simulink model "bh_6dof_quat_integrate"  (R2019b)
settings: Solver=ode45  StartTime=0.0  StopTime=200  FixedStep=0.001  EnableMultiTasking=on
undefined symbols (not defined in the file or in its folder): P_elec, P_mot, P_one_prop, P_rot, P_veh, sigbuilder_block
libraries: bh_6dof_LIBRARY x23, simulink_extras x20, simulink x16
(part 1 of 3)
settings Model: Creator=bhorton  LastModifiedBy=bhorton
settings SolverCC: ZeroCrossAlgorithm=Adaptive  SolverOrder=4
settings DataIOCC: SaveOutput=off  SignalLogging=off  DSMLogging=off  VisualizeSimOutput=off  SaveTime=off  ReturnWorkspaceOutputs=off
settings OptimizationCC: LifeSpan=inf
settings DebuggingCC: AllowSymbolicDim=off  SFUnexpectedBacktrackingDiag=warning  SFNoUnconditionalDefaultTransitionDiag=warning  ArithmeticOperatorsInVariantConditions=warning
settings ModelReferenceCC: PropagateSignalLabelsOutOfModel=off
settings SFSimCC: SimUseLocalCustomCode=off  CustomCodeUndefinedFunction=UseInterfaceOnly
settings RTWCC: RTWUseLocalCustomCode=off
settings CodeAppCC: StateflowObjectComments=on
settings GRTTargetCC: TargetLangStandard=C89/C90 (ANSI)
settings ConfigComp: CovMetricSettings=dw  CovHtmlReporting=on  CovSaveCumulativeToWorkspaceVar=on  CovSaveSingleToWorkspaceVar=on  CovExternalEMLEnable=off

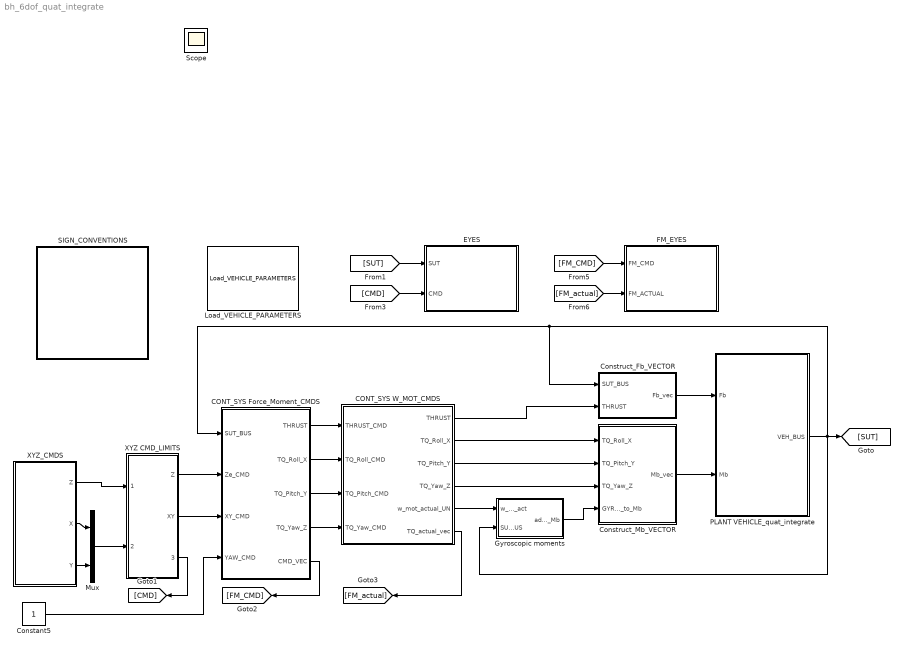
== system bh_6dof_quat_integrate ==
  CONT_SYS Force_Moment_CMDS : Subsystem
  CONT_SYS W_MOT_CMDS : Subsystem
  Constant5 : Constant
  Construct_Fb_VECTOR : Subsystem
  Construct_Mb_VECTOR : Subsystem
  EYES : Subsystem
      mask Display: image('bh_PIC_SCOPE.jpg');
  FM_EYES : Subsystem
      mask Display: image('bh_PIC_SCOPE.jpg');
  Gyroscopic moments : Subsystem
  Load_VEHICLE_PARAMETERS : bh_6dof_LIBRARY/MODELS/Load_VEHICLE_PARAMETERS  SystemSampleTime=-1  Latency=0  AutoFrameSizeCalculation=off
  Mux : Mux  Inputs=2
  PLANT VEHICLE_quat_integrate : Subsystem
  SIGN_CONVENTIONS : Subsystem
  XYZ CMD_LIMITS : Subsystem
  XYZ_CMDS : Subsystem  Tag=STV Subsys  LoadFcn=sigbuilder_block('load');  StartFcn=sigbuilder_block('start');  StopFcn=sigbuilder_block('stop');  ClipboardFcn=sigbuilder_block('clipboard');  mask(Sigbuilder block){tuvar=[0:10]}
      mask help: Simulink:masks:SigbuilderBlock_MD
      mask init:
      | if ~strcmp(get_param(bdroot(gcbh),'SimulationStatus'),'stopped') tuvar = sigbuilder_block('maskInit'); end
      settings: CopyFcn=sigbuilder_block('copy');  DeleteFcn=sigbuilder_block('delete');  ModelCloseFcn=sigbuilder_block('modelClose');  PreSaveFcn=sigbuilder_block('preSave');  PauseFcn=sigbuilder_block('pause');  ContinueFcn=sigbuilder_block('continue');  NameChangeFcn=sigbuilder_block('namechange');  OpenFcn=sigbuilder_block('open',[189 32.25 551.25 400.5 ]);  CloseFcn=sigbuilder_block('close');
      mask Display: plot(0, 0, 100, 100,[2, 2, 32, 32, 2], [68, 8, 8, 68, 68],[32, 2], [38, 38], [32, 19, 2],[53, 60, 44], [32, 17, 17, 2],[16, 16, 31, 31]);txt = getActiveGroup(gcbh);text(2, 100, txt,'verticalAlignment', 'top');
  Scope : Scope
  wires:
  Construct_Fb_VECTOR/1(Fb_vec) -> PLANT VEHICLE_quat_integrate/1(Fb)
  Construct_Mb_VECTOR/1(Mb_vec) -> PLANT VEHICLE_quat_integrate/2(Mb)
  CONT_SYS Force_Moment_CMDS/1(THRUST) -> CONT_SYS W_MOT_CMDS/1(THRUST_CMD)
  Constant5/1 -> CONT_SYS Force_Moment_CMDS/4(YAW_CMD)
  XYZ_CMDS/1(Z) -> XYZ CMD_LIMITS/1(Z_CMD)
  [SUT] -> EYES/1(SUT)
  [CMD] -> EYES/2(CMD)
  XYZ CMD_LIMITS/3(CMD_BUS) -> [CMD]
  XYZ CMD_LIMITS/2(XY) -> CONT_SYS Force_Moment_CMDS/3(XY_CMD)
  XYZ CMD_LIMITS/1(Z) -> CONT_SYS Force_Moment_CMDS/2(Ze_CMD)
  Mux/1 -> XYZ CMD_LIMITS/2(XY_CMD)
  XYZ_CMDS/3(Y) -> Mux/2
  XYZ_CMDS/2(X) -> Mux/1
  CONT_SYS W_MOT_CMDS/1(THRUST) -> Construct_Fb_VECTOR/2(THRUST)
  CONT_SYS W_MOT_CMDS/2(TQ_Roll_X) -> Construct_Mb_VECTOR/1(TQ_Roll_X)
  CONT_SYS W_MOT_CMDS/3(TQ_Pitch_Y) -> Construct_Mb_VECTOR/2(TQ_Pitch_Y)
  CONT_SYS W_MOT_CMDS/4(TQ_Yaw_Z) -> Construct_Mb_VECTOR/3(TQ_Yaw_Z)
  CONT_SYS W_MOT_CMDS/6(TQ_actual_vec) -> [FM_actual]
  [FM_CMD] -> FM_EYES/1(FM_CMD)
  [FM_actual] -> FM_EYES/2(FM_ACTUAL)
  PLANT VEHICLE_quat_integrate/1(VEH_BUS) -> Gyroscopic moments/2(SUT_BUS), Construct_Fb_VECTOR/1(SUT_BUS), CONT_SYS Force_Moment_CMDS/1(SUT_BUS), [SUT]
  Gyroscopic moments/1(add_to_Mb) -> Construct_Mb_VECTOR/4(GYRO_add_to_Mb)
  CONT_SYS W_MOT_CMDS/5(w_mot_actual_UN) -> Gyroscopic moments/1(w_mot_act)
  CONT_SYS Force_Moment_CMDS/2(TQ_Roll_X) -> CONT_SYS W_MOT_CMDS/2(TQ_Roll_CMD)
  CONT_SYS Force_Moment_CMDS/3(TQ_Pitch_Y) -> CONT_SYS W_MOT_CMDS/3(TQ_Pitch_CMD)
  CONT_SYS Force_Moment_CMDS/4(TQ_Yaw_Z) -> CONT_SYS W_MOT_CMDS/4(TQ_Yaw_CMD)
  CONT_SYS Force_Moment_CMDS/5(CMD_VEC) -> [FM_CMD]

== system bh_6dof_quat_integrate/CONT_SYS Force_Moment_CMDS ==
  SUT_BUS : Inport
  Ze_CMD : Inport  Port=2
  XY_CMD : Inport  Port=3
  YAW_CMD : Inport  Port=4
  Constant3 : Constant  Value=P_veh.mass
  FM_CMD_LIMITS : Subsystem
  Gain : Gain  Gain=9.81
  PITCH_and_ROLL_CONT : Subsystem
  Sum2 : Sum  Inputs=++|
  YAW_CONT : Subsystem
  Z_CONT : Subsystem
  THRUST : Outport
  TQ_Roll_X : Outport  Port=2
  TQ_Pitch_Y : Outport  Port=3
  TQ_Yaw_Z : Outport  Port=4
  CMD_VEC : Outport  Port=5
  wires:
  SUT_BUS/1 -> YAW_CONT/2(SUT_BUS), PITCH_and_ROLL_CONT/2(SUT_BUS), Z_CONT/2(SUT_BUS)
  Ze_CMD/1 -> Z_CONT/1(Ze_CMD)
  XY_CMD/1 -> PITCH_and_ROLL_CONT/1(XY_CMD)
  YAW_CMD/1 -> YAW_CONT/1(Yaw_CMD)
  Z_CONT/1(THRUST) -> Sum2/2
  PITCH_and_ROLL_CONT/1(TQ_Roll) -> FM_CMD_LIMITS/2(TQ_Roll)
  PITCH_and_ROLL_CONT/2(TQ_Pitch) -> FM_CMD_LIMITS/3(TQ_Pitch)
  Sum2/1 -> FM_CMD_LIMITS/1(T_CMD)
  YAW_CONT/1(TQ_Yaw) -> FM_CMD_LIMITS/4(TQ_Yaw)
  FM_CMD_LIMITS/1(THRUST) -> THRUST/1
  FM_CMD_LIMITS/2(TQ_Roll_X) -> TQ_Roll_X/1
  FM_CMD_LIMITS/3(TQ_Pitch_Y) -> TQ_Pitch_Y/1
  FM_CMD_LIMITS/4(TQ_Yaw_Z) -> TQ_Yaw_Z/1
  FM_CMD_LIMITS/5(CMD_VEC) -> CMD_VEC/1
  Gain/1 -> Sum2/1
  Constant3/1 -> Gain/1

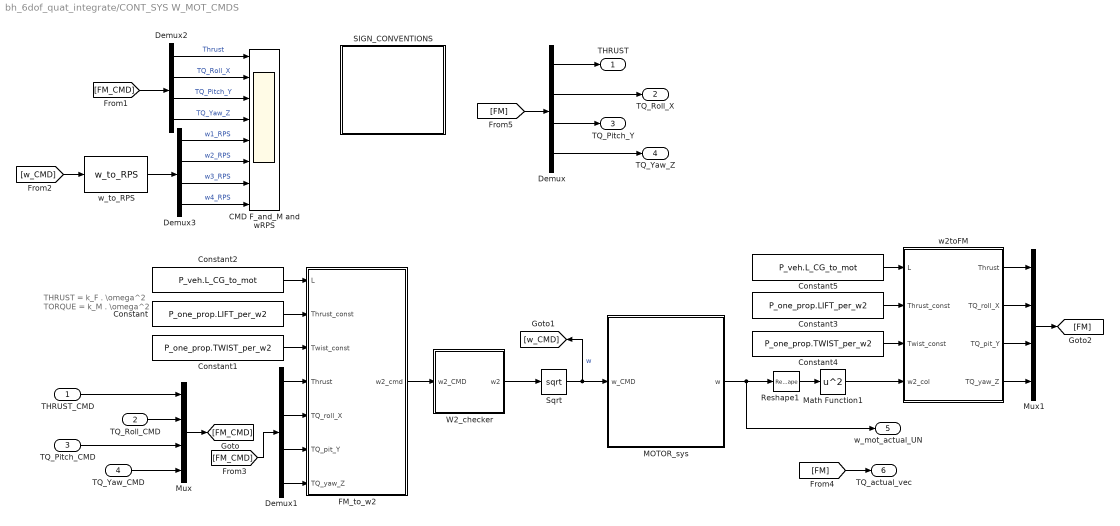
== system bh_6dof_quat_integrate/CONT_SYS W_MOT_CMDS ==
  note: THRUST = k_F . \omega^2
      |
      | TORQUE = k_M . \omega^2
  THRUST_CMD : Inport
  TQ_Roll_CMD : Inport  Port=2
  TQ_Pitch_CMD : Inport  Port=3
  TQ_Yaw_CMD : Inport  Port=4
  CMD F_and_M and wRPS : Scope  NumInputPorts=8
  Constant : Constant  Value=P_one_prop.LIFT_per_w2
  Constant1 : Constant  Value=P_one_prop.TWIST_per_w2
  Constant2 : Constant  Value=P_veh.L_CG_to_mot
  Constant3 : Constant  Value=P_one_prop.LIFT_per_w2
  Constant4 : Constant  Value=P_one_prop.TWIST_per_w2
  Constant5 : Constant  Value=P_veh.L_CG_to_mot
  Demux{,1..3} (4 alike) : Demux
  FM_to_w2 : MATLAB Function  TreatAsAtomicUnit=on
  MOTOR_sys : Subsystem
      mask Display: image('bh_PIC_MOTOR.jpg');
  Math Function1 : Math  Operator=square  SaturateOnIntegerOverflow=on
  Mux : Mux
  Mux1 : Mux
  Reshape1 : Reshape  OutputDimensionality=Column vector (2-D)
  SIGN_CONVENTIONS : Subsystem
  Sqrt : Sqrt  SaturateOnIntegerOverflow=on
  W2_checker : Subsystem
  w2toFM : MATLAB Function  TreatAsAtomicUnit=on
  w_to_RPS : bh_6dof_LIBRARY/MODELS/w_to_RPS  SystemSampleTime=-1  Latency=0  AutoFrameSizeCalculation=off
  THRUST : Outport
  TQ_Roll_X : Outport  Port=2
  TQ_Pitch_Y : Outport  Port=3
  TQ_Yaw_Z : Outport  Port=4
  w_mot_actual_UN : Outport  Port=5
  TQ_actual_vec : Outport  Port=6
  wires:
  Constant1/1 -> FM_to_w2/3(Twist_const)
  Constant/1 -> FM_to_w2/2(Thrust_const)
  Constant2/1 -> FM_to_w2/1(L)
  FM_to_w2/1(w2_cmd) -> W2_checker/1(w2_CMD)
  Sqrt/1 -> MOTOR_sys/1(w_CMD), [w_CMD]  "w"
  W2_checker/1(w2) -> Sqrt/1
  Demux1/1 -> FM_to_w2/4(Thrust)
  Demux1/2 -> FM_to_w2/5(TQ_roll_X)
  Demux1/3 -> FM_to_w2/6(TQ_pit_Y)
  Demux1/4 -> FM_to_w2/7(TQ_yaw_Z)
  THRUST_CMD/1 -> Mux/1
  TQ_Roll_CMD/1 -> Mux/2
  TQ_Pitch_CMD/1 -> Mux/3
  TQ_Yaw_CMD/1 -> Mux/4
  Mux/1 -> [FM_CMD]
  [FM_CMD] -> Demux1/1
  Demux2/1 -> CMD F_and_M and wRPS/1  "Thrust"
  Demux2/2 -> CMD F_and_M and wRPS/2  "TQ_Roll_X"
  Demux2/3 -> CMD F_and_M and wRPS/3  "TQ_Pitch_Y"
  Demux2/4 -> CMD F_and_M and wRPS/4  "TQ_Yaw_Z"
  Demux3/2 -> CMD F_and_M and wRPS/6  "w2_RPS"
  Demux3/1 -> CMD F_and_M and wRPS/5  "w1_RPS"
  Demux3/4 -> CMD F_and_M and wRPS/8  "w4_RPS"
  Demux3/3 -> CMD F_and_M and wRPS/7  "w3_RPS"
  [FM_CMD] -> Demux2/1
  w_to_RPS/1 -> Demux3/1
  [w_CMD] -> w_to_RPS/1
  Constant3/1 -> w2toFM/2(Thrust_const)
  Constant4/1 -> w2toFM/3(Twist_const)
  Constant5/1 -> w2toFM/1(L)
  w2toFM/1(Thrust) -> Mux1/1
  w2toFM/2(TQ_roll_X) -> Mux1/2
  w2toFM/3(TQ_pit_Y) -> Mux1/3
  w2toFM/4(TQ_yaw_Z) -> Mux1/4
  Mux1/1 -> [FM]
  Demux/1 -> THRUST/1
  Demux/2 -> TQ_Roll_X/1
  Demux/4 -> TQ_Yaw_Z/1
  Demux/3 -> TQ_Pitch_Y/1
  [FM] -> Demux/1
  Reshape1/1 -> Math Function1/1
  Math Function1/1 -> w2toFM/4(w2_col)
  [FM] -> TQ_actual_vec/1
  MOTOR_sys/1(w) -> Reshape1/1, w_mot_actual_UN/1

== system bh_6dof_quat_integrate/Construct_Fb_VECTOR ==
  SUT_BUS : Inport
  THRUST : Inport  Port=2
  Bus Selector1 : BusSelector  OutputSignals=DCM_bRg
  Constant1 : Constant  Value=0
  Gravity_G_to_B : Subsystem
  Mux : Mux  Inputs=3
  Reshape : Reshape  OutputDimensionality=Column vector (2-D)
  Sum : Sum  Inputs=++|
  Fb_vec : Outport
  wires:
  Mux/1 -> Reshape/1
  Sum/1 -> Fb_vec/1
  SUT_BUS/1 -> Bus Selector1/1
  THRUST/1 -> Mux/3  "THRUST"
  Constant1/1 -> Mux/2, Mux/1
  Bus Selector1/1 -> Gravity_G_to_B/1(bRg)  "<DCM_bRg>"
  Gravity_G_to_B/1(Fb_gravity) -> Sum/1
  Reshape/1 -> Sum/2

== system bh_6dof_quat_integrate/Construct_Mb_VECTOR ==
  TQ_Roll_X : Inport
  TQ_Pitch_Y : Inport  Port=2
  TQ_Yaw_Z : Inport  Port=3
  GYRO_add_to_Mb : Inport  Port=4
  Mux1 : Mux  Inputs=3
  Reshape : Reshape  OutputDimensionality=Column vector (2-D)
  Reshape1 : Reshape  OutputDimensionality=Column vector (2-D)
  Sum : Sum  Inputs=+|+
  Mb_vec : Outport
  wires:
  TQ_Yaw_Z/1 -> Mux1/3
  TQ_Pitch_Y/1 -> Mux1/2
  TQ_Roll_X/1 -> Mux1/1
  Mux1/1 -> Reshape/1
  Sum/1 -> Reshape1/1
  Reshape/1 -> Sum/1
  GYRO_add_to_Mb/1 -> Sum/2
  Reshape1/1 -> Mb_vec/1

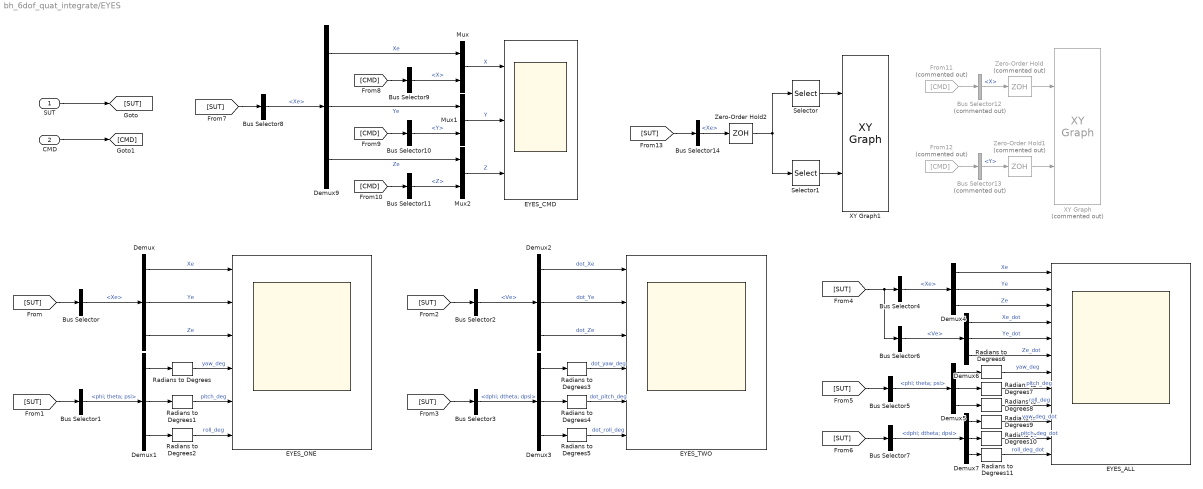
== system bh_6dof_quat_integrate/EYES ==
  SUT : Inport
  CMD : Inport  Port=2
  Bus Selector{,4,8,14} (4 alike) : BusSelector  OutputSignals=Xe
  Bus Selector1 : BusSelector  OutputSignals=phi; theta; psi
  Bus Selector10 : BusSelector  OutputSignals=Y
  Bus Selector11 : BusSelector  OutputSignals=Z
  Bus Selector12 : BusSelector  Commented=on  OutputSignals=X
  Bus Selector13 : BusSelector  Commented=on  OutputSignals=Y
  Bus Selector2 : BusSelector  OutputSignals=Ve
  Bus Selector3 : BusSelector  OutputSignals=dphi; dtheta; dpsi
  Bus Selector5 : BusSelector  OutputSignals=phi; theta; psi
  Bus Selector6 : BusSelector  OutputSignals=Ve
  Bus Selector7 : BusSelector  OutputSignals=dphi; dtheta; dpsi
  Bus Selector9 : BusSelector  OutputSignals=X
  Demux{,1..7,9} (9 alike) : Demux  Outputs=3
  EYES_ALL : Scope  NumInputPorts=12
  EYES_CMD : Scope  NumInputPorts=3
  EYES_ONE : Scope  NumInputPorts=6
  EYES_TWO : Scope  NumInputPorts=6
  From11 : From  Commented=on  GotoTag=CMD
  From12 : From  Commented=on  GotoTag=CMD
  Mux : Mux  Inputs=2
  Mux1 : Mux  Inputs=2
  Mux2 : Mux  Inputs=2
  Radians to Degrees{,1..11} (12 alike) : simulink_extras/Transformations/Radians to Degrees
  Selector : Selector  InputPortWidth=3  IndexOptions=Index vector (dialog)  Indices=1  OutputSizes=1
  Selector1 : Selector  InputPortWidth=3  IndexOptions=Index vector (dialog)  Indices=2  OutputSizes=1
  XY Graph : simulink/Sinks/XY Graph  Commented=on  xmin=-1  xmax=30  ymin=-1  ymax=35  st=-1
  XY Graph1 : simulink/Sinks/XY Graph  xmin=-1  xmax=30  ymin=-1  ymax=35  st=-1
  Zero-Order Hold : ZeroOrderHold  Commented=on  SampleTime=0.1
  Zero-Order Hold1 : ZeroOrderHold  Commented=on  SampleTime=0.1
  Zero-Order Hold2 : ZeroOrderHold  SampleTime=0.1
  wires:
  SUT/1 -> [SUT]
  [SUT] -> Bus Selector/1
  Demux/2 -> EYES_ONE/2  "Ye"
  Demux/3 -> EYES_ONE/3  "Ze"
  Demux/1 -> EYES_ONE/1  "Xe"
  Bus Selector/1 -> Demux/1  "<Xe>"
  Bus Selector1/1 -> Demux1/1  "<phi; theta; psi>"
  [SUT] -> Bus Selector1/1
  Demux1/1 -> Radians to Degrees/1
  Radians to Degrees/1 -> EYES_ONE/4  "yaw_deg"
  Radians to Degrees1/1 -> EYES_ONE/5  "pitch_deg"
  Radians to Degrees2/1 -> EYES_ONE/6  "roll_deg"
  Demux1/3 -> Radians to Degrees2/1
  Demux1/2 -> Radians to Degrees1/1
  [SUT] -> Bus Selector2/1
  Demux2/2 -> EYES_TWO/2  "dot_Ye"
  Demux2/3 -> EYES_TWO/3  "dot_Ze"
  Demux2/1 -> EYES_TWO/1  "dot_Xe"
  Bus Selector2/1 -> Demux2/1  "<Ve>"
  Bus Selector3/1 -> Demux3/1  "<dphi; dtheta; dpsi>"
  [SUT] -> Bus Selector3/1
  Demux3/1 -> Radians to Degrees3/1
  Radians to Degrees3/1 -> EYES_TWO/4  "dot_yaw_deg"
  Radians to Degrees4/1 -> EYES_TWO/5  "dot_pitch_deg"
  Radians to Degrees5/1 -> EYES_TWO/6  "dot_roll_deg"
  Demux3/3 -> Radians to Degrees5/1
  Demux3/2 -> Radians to Degrees4/1
  [SUT] -> Bus Selector6/1, Bus Selector4/1
  Demux4/2 -> EYES_ALL/2  "Ye"
  Demux4/3 -> EYES_ALL/3  "Ze"
  Demux4/1 -> EYES_ALL/1  "Xe"
  Bus Selector4/1 -> Demux4/1  "<Xe>"
  Bus Selector5/1 -> Demux5/1  "<phi; theta; psi>"
  [SUT] -> Bus Selector5/1
  Demux5/1 -> Radians to Degrees6/1
  Demux6/1 -> EYES_ALL/4  "Xe_dot"
  Demux6/2 -> EYES_ALL/5  "Ye_dot"
  Demux6/3 -> EYES_ALL/6  "Ze_dot"
  Demux5/3 -> Radians to Degrees8/1
  Demux5/2 -> Radians to Degrees7/1
  Bus Selector6/1 -> Demux6/1  "<Ve>"
  Radians to Degrees6/1 -> EYES_ALL/7  "yaw_deg"
  Radians to Degrees7/1 -> EYES_ALL/8  "pitch_deg"
  Radians to Degrees8/1 -> EYES_ALL/9  "roll_deg"
  Bus Selector7/1 -> Demux7/1  "<dphi; dtheta; dpsi>"
  [SUT] -> Bus Selector7/1
  Demux7/1 -> Radians to Degrees9/1
  Demux7/2 -> Radians to Degrees10/1
  Demux7/3 -> Radians to Degrees11/1
  Radians to Degrees9/1 -> EYES_ALL/10  "yaw_deg_dot"
  Radians to Degrees10/1 -> EYES_ALL/11  "pitch_deg_dot"
  Radians to Degrees11/1 -> EYES_ALL/12  "roll_deg_dot"
  CMD/1 -> [CMD]
  [SUT] -> Bus Selector8/1
  Demux9/2 -> Mux1/1  "Ye"
  Demux9/1 -> Mux/1  "Xe"
  Bus Selector8/1 -> Demux9/1  "<Xe>"
  Mux/1 -> EYES_CMD/1  "X"
  Mux1/1 -> EYES_CMD/2  "Y"
  Mux2/1 -> EYES_CMD/3  "Z"
  Demux9/3 -> Mux2/1  "Ze"
  [CMD] -> Bus Selector9/1
  Bus Selector9/1 -> Mux/2  "<X>"
  [CMD] -> Bus Selector10/1
  Bus Selector10/1 -> Mux1/2  "<Y>"
  [CMD] -> Bus Selector11/1
  Bus Selector11/1 -> Mux2/2  "<Z>"
  From11/1 -> Bus Selector12/1
  Bus Selector12/1 -> Zero-Order Hold/1  "<X>"
  From12/1 -> Bus Selector13/1
  Bus Selector13/1 -> Zero-Order Hold1/1  "<Y>"
  Zero-Order Hold/1 -> XY Graph/1
  Zero-Order Hold1/1 -> XY Graph/2
  [SUT] -> Bus Selector14/1
  Bus Selector14/1 -> Zero-Order Hold2/1  "<Xe>"
  Zero-Order Hold2/1 -> Selector1/1, Selector/1
  Selector1/1 -> XY Graph1/2
  Selector/1 -> XY Graph1/1

== system bh_6dof_quat_integrate/FM_EYES ==
  FM_CMD : Inport
  FM_ACTUAL : Inport  Port=2
  FM CMD vs Actual : Scope  NumInputPorts=4
  FM_Mux : Subsystem
  SIGN_CONVENTIONS : Subsystem
  wires:
  FM_CMD/1 -> [FM_CMD]
  [FM_CMD] -> FM_Mux/1(FM_CMD)
  [FM] -> FM_Mux/2(FM)
  FM_Mux/1(Y1) -> FM CMD vs Actual/1  "Thrust"
  FM_Mux/2(Y2) -> FM CMD vs Actual/2  "TQ_Roll_X"
  FM_Mux/3(w3) -> FM CMD vs Actual/3  "TQ_Pitch_Y"
  FM_Mux/4(Y4) -> FM CMD vs Actual/4  "TQ_Yaw_Z"
  FM_ACTUAL/1 -> [FM]

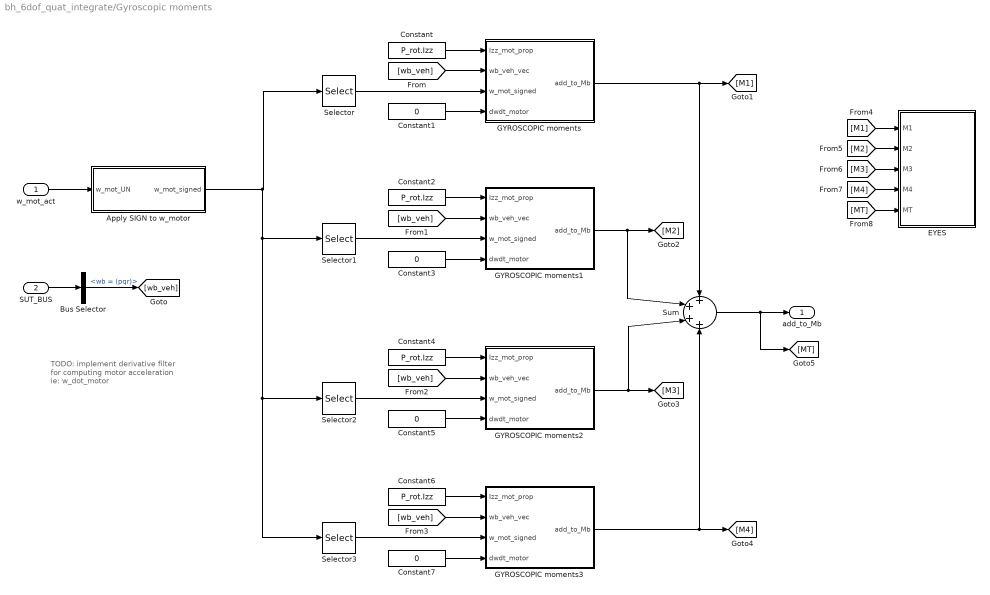
== system bh_6dof_quat_integrate/Gyroscopic moments ==
  note: TODO:
      | implement derivative filter
      | for computing motor acceleration
      | ie: w_dot_motor
  w_mot_act : Inport
  SUT_BUS : Inport  Port=2
  Apply SIGN to w_motor : Subsystem
  Bus Selector : BusSelector  OutputSignals=wb = (pqr)
  Constant{,2,4,6} (4 alike) : Constant  Value=P_rot.Izz  VectorParams1D=off
  Constant{1,3,5,7} (4 alike) : Constant  Value=0  VectorParams1D=off
  EYES : Subsystem
  GYROSCOPIC moments : Subsystem
  GYROSCOPIC moments1 : Subsystem
  GYROSCOPIC moments2 : Subsystem
  GYROSCOPIC moments3 : Subsystem
  Selector : Selector  InputPortWidth=4  IndexOptions=Index vector (dialog)  Indices=1  OutputSizes=1
  Selector1 : Selector  InputPortWidth=4  IndexOptions=Index vector (dialog)  Indices=2  OutputSizes=1
  Selector2 : Selector  InputPortWidth=4  IndexOptions=Index vector (dialog)  Indices=3  OutputSizes=1
  Selector3 : Selector  InputPortWidth=4  IndexOptions=Index vector (dialog)  Indices=4  OutputSizes=1
  Sum : Sum  Inputs=+|+|+|+
  add_to_Mb : Outport
  wires:
  SUT_BUS/1 -> Bus Selector/1
  w_mot_act/1 -> Apply SIGN to w_motor/1(w_mot_UN)
  Bus Selector/1 -> [wb_veh]  "<wb = (pqr)>"
  [wb_veh] -> GYROSCOPIC moments/2(wb_veh_vec)
  Constant1/1 -> GYROSCOPIC moments/4(dwdt_motor)
  Constant/1 -> GYROSCOPIC moments/1(Izz_mot_prop)
  Selector/1 -> GYROSCOPIC moments/3(w_mot_signed)
  Apply SIGN to w_motor/1(w_mot_signed) -> Selector1/1, Selector2/1, Selector3/1, Selector/1
  [wb_veh] -> GYROSCOPIC moments1/2(wb_veh_vec)
  Constant3/1 -> GYROSCOPIC moments1/4(dwdt_motor)
  Constant2/1 -> GYROSCOPIC moments1/1(Izz_mot_prop)
  Selector1/1 -> GYROSCOPIC moments1/3(w_mot_signed)
  [wb_veh] -> GYROSCOPIC moments2/2(wb_veh_vec)
  Constant5/1 -> GYROSCOPIC moments2/4(dwdt_motor)
  Constant4/1 -> GYROSCOPIC moments2/1(Izz_mot_prop)
  Selector2/1 -> GYROSCOPIC moments2/3(w_mot_signed)
  [wb_veh] -> GYROSCOPIC moments3/2(wb_veh_vec)
  Constant7/1 -> GYROSCOPIC moments3/4(dwdt_motor)
  Constant6/1 -> GYROSCOPIC moments3/1(Izz_mot_prop)
  Selector3/1 -> GYROSCOPIC moments3/3(w_mot_signed)
  GYROSCOPIC moments/1(add_to_Mb) -> [M1], Sum/1
  GYROSCOPIC moments3/1(add_to_Mb) -> [M4], Sum/4
  GYROSCOPIC moments1/1(add_to_Mb) -> [M2], Sum/2
  GYROSCOPIC moments2/1(add_to_Mb) -> [M3], Sum/3
  Sum/1 -> [MT], add_to_Mb/1
  [MT] -> EYES/5(MT)
  [M4] -> EYES/4(M4)
  [M3] -> EYES/3(M3)
  [M2] -> EYES/2(M2)
  [M1] -> EYES/1(M1)

== system bh_6dof_quat_integrate/PLANT VEHICLE_quat_integrate ==
  Fb : Inport
  Mb : Inport  Port=2
  Bus Creator : BusCreator  Inputs=10
  bh_6DOF_quat_integrate : Subsystem  mask(bh_6DOF EoM (Body Axis) QUATERNION approach){inertia_0=P_veh.I, mass_0=P_veh.mass, xme_0=P_veh.Xe_init, Vm_0=P_veh.Vb_init, pm_0=P_veh.wb_init, eul_0=P_veh.eul_init}
      mask prompts: inertia_0 "Vehicle Inertia, [kg.m^2]"; mass_0 "Vehicle Mass, [kg]"; xme_0 "Initial position in inertial axes [Xe,Ye,Ze], [m]"; Vm_0 "Initial velocity in body axes [U,v,w], [m/sec]"; pm_0 "Initial body rotation rates [p,q,r], [rad/sec]"; eul_0 "Initial Euler orientation [yaw, pitch, roll], [rad]"
      mask init:
      | OBJ_q = bh_rots_PKG.bh_quat_rot_CLS();
      | q_0   = OBJ_q.calc_q_from_YPR(eul_0(1), eul_0(2), eul_0(3) );
      mask DialogControl DescTextVar Prompt: Implementation of a 6-DOF rigid body equations of motion.
      mask DialogControl Control16 Prompt: QUATERNIONS are used to describe angular pose. We integrate the QUATERNION derivative to calculate q and then use the QUATERNION to compute the Euler angles.
      mask DialogControl Container16 Prompt: PASSIVE rotation sequence
      mask DialogControl Control22 Prompt: The co-ordinate transformation that converts the components of a
      mask DialogControl Control23 Prompt: G-frame vector into its components in the B-frame, is:
      mask DialogControl Control51 Prompt: (Add text here)
      mask DialogControl Control24 Prompt: vb = pR3X(psi) * pR2Y(theta) * pR1Z(phi) * vg
      mask DialogControl Control25 Prompt: vb = bRg * vg
      mask DialogControl Control53 Prompt: You can READ more about PASSIVE rotations, HERE.
      mask DialogControl Control53 Callback: winopen('CONCEPT_PASSIVE_rotations.pdf')
      mask DialogControl Container22 Prompt: ACTIVE rotation sequence
      mask DialogControl Control26 Prompt: To actively reposition (ie: rotate) a B-frame that is initially coincident
      mask DialogControl Control27 Prompt: with the inertial G-frame, into a new pose, we would:
      mask DialogControl Control49 Prompt: (Add text here)
      mask DialogControl Control28 Prompt: vg = inv(pR1Z(phi)) * inv(pR2Y(theta)) * inv(pR3X(psi)) * vb
      mask DialogControl Control46 Prompt: (Add text here)
      mask DialogControl Control30 Prompt: If we define:    aR( ) == inv( pR()  ),  then we can write the above as:
      mask DialogControl Control31 Prompt: (Add text here)
      mask DialogControl Control32 Prompt: vg = aR1Z(phi) * aR2Y(theta) * aR3(psi) * vb
      mask DialogControl Control40 Prompt: You can READ more about ACTIVE rotations, HERE.
      mask DialogControl Control40 Callback: winopen('CONCEPT_ACTIVE_rotations.pdf')
      mask DialogControl Container4 Prompt: Parameters
      mask DialogControl Control11 Prompt: ATTENTION:  note the order of the angles in the list above.
      mask DialogControl Control12 Prompt: This is DIFFERENT to the order used in the Aerospace blockset.
      mask DialogControl Container6 Prompt: DOC
      mask DialogControl Control6 Prompt: In this EULER angle implementation we define the
      mask DialogControl Control7 Prompt: following sequence that rotates a G-frame
      mask DialogControl Control8 Prompt: into a B-frame:
      mask DialogControl Control9_copy Prompt: 1.)  R1Z  : a local rotation about the Z axis by phi, (YAW)
      mask DialogControl Control9_copy_copy Prompt: 2.)  R2Y  : a local rotation about the Y axis by theta, (PITCH)
      mask DialogControl Control17 Prompt: 3.)  R3X  : a local rotation about the X axis by psi, (ROLL)
      mask DialogControl Container8 Prompt: EoM  - part 1
      mask DialogControl Control18 Prompt: The translational Rigid body Equations of motion are:
      mask DialogControl Container9 Prompt: EoM - part 2
      mask DialogControl Control20 Prompt: The rotational Rigid body Equations of motion are
      mask Display:
      | port_label('input',1,'{{Fb_{xyz}} (N)}','texmode','on');
      | port_label('input',2,'{{Mb_{xyz}} (N-m)}','texmode','on');
      | port_label('output',1,'{V_e (m/s)}','texmode','on');
      | port_label('output',2,'{X_e (m)}','texmode','on');
      | port_label('output',3,'{\Phi_{Z1} \theta_{Y2} \Psi_{X3} (rad)}','texmode','on');
      | port_label('output',4,'{DCM bRg }','texmode','on');
      | port_label('output',5,'{V_b (m/s)}','texmode','on');
      | port_label('output',6,'{{\omega_b (rad/s)}}','texmode','on');
      | port_label('output',7,'{{d\omega_b/dt}}','texmode','on');
      | port_label('output',8,'{A_b (m/s^2)}','texmode','on');
      | port_label('output',9,'{d\Phi_{Z1} d\theta_{Y2} d\Psi_{X3} (rad/sec)}','texmode','on');
      | port_label('output',10,'{q = [q_0, q_X, q_Y, q_Z]}','texmode','on');
      | 
      | text(0.5,0.7248,'QUATERNION\nintegration','horizontalAlignment','center')
      | 
      | text(0.5,0.3112,'Fixed\nMass','horizontalAlignment','center')
  VEH_BUS : Outport
  wires:
  Fb/1 -> bh_6DOF_quat_integrate/1(Forces)
  Mb/1 -> bh_6DOF_quat_integrate/2(Moments)
  bh_6DOF_quat_integrate/3(Euler) -> Bus Creator/3  "phi; theta; psi"
  bh_6DOF_quat_integrate/2(Xe) -> Bus Creator/2  "Xe"
  bh_6DOF_quat_integrate/1(Ve) -> Bus Creator/1  "Ve"
  bh_6DOF_quat_integrate/4(bRg (DCM)) -> Bus Creator/4  "DCM_bRg"
  bh_6DOF_quat_integrate/8(Ab) -> Bus Creator/8  "Ab"
  bh_6DOF_quat_integrate/7(pdot,qdot,rdot) -> Bus Creator/7  "wb_dot = (pdot;qdot;rdot)"
  bh_6DOF_quat_integrate/5(Vb) -> Bus Creator/5  "Vb"
  bh_6DOF_quat_integrate/6(p,q,r) -> Bus Creator/6  "wb = (pqr)"
  bh_6DOF_quat_integrate/9(Euler_rates) -> Bus Creator/9  "dphi; dtheta; dpsi"
  Bus Creator/1 -> VEH_BUS/1
  bh_6DOF_quat_integrate/10(q) -> Bus Creator/10  "q"

== system bh_6dof_quat_integrate/SIGN_CONVENTIONS ==

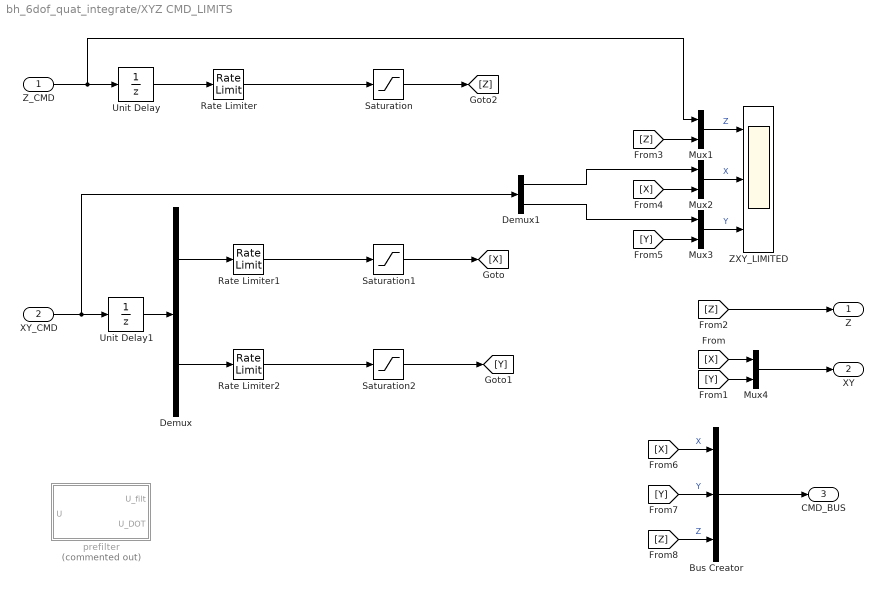
== system bh_6dof_quat_integrate/XYZ CMD_LIMITS ==
  Z_CMD : Inport
  XY_CMD : Inport  Port=2
  Bus Creator : BusCreator  Inputs=3
  Demux : Demux  Outputs=2
  Demux1 : Demux  Outputs=2
  Mux{1..4} (4 alike) : Mux  Inputs=2
  Rate Limiter : RateLimiter  RisingSlewLimit=2  FallingSlewLimit=-2
      settings: AttributesFormatString=|
      | Rising_rate = %<RisingSlewLimit>
      | Falling_rate = %<FallingSlewLimit>
  Rate Limiter1 : RateLimiter  RisingSlewLimit=3  FallingSlewLimit=-3
      settings: AttributesFormatString=|
      | Rising_rate = %<RisingSlewLimit>
      | Falling_rate = %<FallingSlewLimit>
  Rate Limiter2 : RateLimiter  RisingSlewLimit=3  FallingSlewLimit=-3
      settings: AttributesFormatString=|
      | Rising_rate = %<RisingSlewLimit>
      | Falling_rate = %<FallingSlewLimit>
  Saturation : Saturate  UpperLimit=500  LowerLimit=0
      settings: AttributesFormatString=|
      | MAX =    %<UpperLimit>
      | MIN = %<LowerLimit>
  Saturation1 : Saturate  UpperLimit=500  LowerLimit=-500
      settings: AttributesFormatString=|
      | MAX =    %<UpperLimit>
      | MIN = %<LowerLimit>
  Saturation2 : Saturate  UpperLimit=500  LowerLimit=-500
      settings: AttributesFormatString=|
      | MAX =    %<UpperLimit>
      | MIN = %<LowerLimit>
  Unit Delay : UnitDelay  SampleTime=0.01  HasFrameUpgradeWarning=on
  Unit Delay1 : UnitDelay  SampleTime=0.01  HasFrameUpgradeWarning=on
  ZXY_LIMITED : Scope  NumInputPorts=3
  prefilter : Subsystem  Commented=on  mask(Derivative Estimation){wn=2*pi*0.5, p=1}
      mask prompts: wn "Natural frequency, wn (rad/sec)"; p "Damping ratio, p"
      mask help:
      | A simple derivative estimator using a 2nd order representation between input and output.
      |
      | The integrators use a discrete FORWARd Euler rule, and a sample time needs to be specified.
      mask init:
      | str1 = sprintf('wn = %.2f', wn);
      | str2 = sprintf('p  = %.2f', p);
      | %str3 = sprintf('dt = %.2f', dt);
      | %str = char(str1,str2,str3);
      | %str3 = sprintf('dt = %.2f', dt);
      | str = char(str1,str2);
      mask Display: disp(str)
  Z : Outport
  XY : Outport  Port=2
  CMD_BUS : Outport  Port=3
  wires:
  XY_CMD/1 -> Demux1/1, Unit Delay1/1
  Demux/1 -> Rate Limiter1/1
  Demux/2 -> Rate Limiter2/1
  Saturation1/1 -> [X]
  Saturation2/1 -> [Y]
  Mux4/1 -> XY/1
  Z_CMD/1 -> Mux1/1, Unit Delay/1
  Rate Limiter/1 -> Saturation/1
  Unit Delay/1 -> Rate Limiter/1
  Unit Delay1/1 -> Demux/1
  Rate Limiter1/1 -> Saturation1/1
  Rate Limiter2/1 -> Saturation2/1
  [X] -> Mux4/1
  [Y] -> Mux4/2
  [Z] -> Z/1
  Saturation/1 -> [Z]
  [Z] -> Mux1/2
  [Y] -> Mux3/2
  Demux1/1 -> Mux2/1
  Demux1/2 -> Mux3/1
  [X] -> Mux2/2
  Mux1/1 -> ZXY_LIMITED/1  "Z"
  Mux2/1 -> ZXY_LIMITED/2  "X"
  Mux3/1 -> ZXY_LIMITED/3  "Y"
  Bus Creator/1 -> CMD_BUS/1
  [Y] -> Bus Creator/2  "Y"
  [X] -> Bus Creator/1  "X"
  [Z] -> Bus Creator/3  "Z"

== system bh_6dof_quat_integrate/XYZ_CMDS ==
  Demux : Demux  Tag=STV Demux  Outputs=3
  FromWs : FromWorkspace  Tag=STV FromWs  VariableName=tuvar  SampleTime=0
      SigBuilderData=|
      | common.afterFinalStr = 'Extrapolate'
      | common.sampleTime = 0
      | dataSet(1).timeRange = [0 200]
      | dataSet(1).name = 'small_steps'
      | dataSet(2).timeRange = [0 200]
      | dataSet(2).name = 'zStairs_xyConstVEL'
      | dataSet(3).timeRange = [0 500]
      | dataSet(3).name = 'sineWaves'
      | dataSet(4).timeRange = [0 200]
      | dataSet(4).name = 'ZERO'
      | dataSet(5).timeRange = [0 200]
      | dataSet(5).name = 'SEARCH_P1'
      | sbobj.Name = 'Signal Builder'
      | sbobj.Groups(1).Name = 'small_steps'
      | sbobj.Groups(1).Signals(1).Name = 'Z'
      | sbobj.Groups(1).Signals(1).XData = [0 10 10.000001 20 20.000001 30 30.000001 55 200]
      | sbobj.Groups(1).Signals(1).YData = [0 0 2 2 2 2 2 2 2]
      | sbobj.Groups(1).Signals(2).Name = 'X'
      | sbobj.Groups(1).Signals(2).XData = [0 10 10.000001 20 20.000001 30 30.000001 55 200]
      | sbobj.Groups(1).Signals(2).YData = [0 0 0 0 3 3 3 3 3]
      | sbobj.Groups(1).Signals(3).Name = 'Y'
      | sbobj.Groups(1).Signals(3).XData = [0 10 10.000001 20 20.000001 30 30.000001 55 200]
      | sbobj.Groups(1).Signals(3).YData = [0 0 0 0 0 0 1 1 1]
      | sbobj.Groups(1).TimeRange = [0 200]
      | sbobj.Groups(2).Name = 'zStairs_xyConstVEL'
      | sbobj.Groups(2).Signals(1).Name = 'Z'
      | sbobj.Groups(2).Signals(1).XData = [0 10 10.000001 20 20.000001 30 30.000001 40 40.000001 55 200]
      | sbobj.Groups(2).Signals(1).YData = [0 0 1 1 2 2 1 1 0 0 0]
      | sbobj.Groups(2).Signals(2).Name = 'X'
      | sbobj.Groups(2).Signals(2).XData = [0 10 10.000001 20 20.000001 30 30.000001 40 40.000001 55 200]
      | sbobj.Groups(2).Signals(2).YData = [0 1 1.0000001 2 2.0000001 3 3.0000001 4 4.0000001 5.5 20]
      | sbobj.Groups(2).Signals(3).Name = 'Y'
      | sbobj.Groups(2).Signals(3).XData = [0 10 10.000001 20 20.000001 30 30.000001 40 40.000001 55 200]
      | sbobj.Groups(2).Signals(3).YData = [0 0.5 0.50000005 1 1.00000005 1.5 1.50000005 2 2.00000005 2.75 10]
      | sbobj.Groups(2).TimeRange = [0 200]
      | sbobj.Groups(3).Name = 'sineWaves'
      | sbobj.Groups(3).Signals(1).Name = 'Z'
      | sbobj.Groups(3).Signals(1).XData = [0 0.1 0.2 0.3 0.4 0.5 0.6 0.7 0.8 0.9 1 1.1 ... (5001 elements, 1x5001)]
      | sbobj.Groups(3).Signals(1).YData = [0 0.0314107325553 0.0627904665622 0.0941082340641 0.125333128258 0.156434333994 0.18738115819 0.218143060119 0.248689681547 0.278990876699 0.309016742004 0.338737645607 ... (5001 elements, 1x5001)]
      | sbobj.Groups(3).Signals(2).Name = 'X'
      | sbobj.Groups(3).Signals(2).XData = [0 0.1 0.2 0.3 0.4 0.5 0.6 0.7 0.8 0.9 1 1.1 ... (5001 elements, 1x5001)]
      | sbobj.Groups(3).Signals(2).YData = [0 0.01 0.02 0.03 0.04 0.05 0.06 0.07 0.08 0.09 0.1 0.11 ... (5001 elements, 1x5001)]
      | sbobj.Groups(3).Signals(3).Name = 'Y'
      | sbobj.Groups(3).Signals(3).XData = [0 0.1 0.2 0.3 0.4 0.5 0.6 0.7 0.8 0.9 1 1.1 ... (5001 elements, 1x5001)]
      | sbobj.Groups(3).Signals(3).YData = [0 0.0157073040455 0.0314107325553 0.04710641095 0.0627904665622 0.0784590295926 0.0941082340641 0.109734218776 0.125333128258 0.140901113717 0.156434333994 0.171928956505 ... (5001 elements, 1x5001)]
      | sbobj.Groups(3).TimeRange = [0 500]
      | sbobj.Groups(4).Name = 'ZERO'
      | sbobj.Groups(4).Signals(1).Name = 'Z'
      | sbobj.Groups(4).Signals(1).XData = [0 200]
      | sbobj.Groups(4).Signals(1).YData = [0 0]
      | sbobj.Groups(4).Signals(2).Name = 'X'
      | sbobj.Groups(4).Signals(2).XData = [0 200]
      | sbobj.Groups(4).Signals(2).YData = [0 0]
      | sbobj.Groups(4).Signals(3).Name = 'Y'
      | sbobj.Groups(4).Signals(3).XData = [0 200]
      | sbobj.Groups(4).Signals(3).YData = [0 0]
      | sbobj.Groups(4).TimeRange = [0 200]
      | sbobj.Groups(5).Name = 'SEARCH_P1'
      | sbobj.Groups(5).Signals(1).Name = 'Z'
      | sbobj.Groups(5).Signals(1).XData = [0 7 27 32 52 57 77 82 102 107 127 132 157 187 200]
      | sbobj.Groups(5).Signals(1).YData = [0 5 5 5 5 5 5 5 5 5 5 5 5 0 0]
      | sbobj.Groups(5).Signals(2).Name = 'X'
      | sbobj.Groups(5).Signals(2).XData = [0 7 27 32 52 57 77 82 102 107 127 132 157 187 200]
      | sbobj.Groups(5).Signals(2).YData = [0 5 25 25 5 5 25 25 5 5 25 25 0 0 0]
      | sbobj.Groups(5).Signals(3).Name = 'Y'
      | sbobj.Groups(5).Signals(3).XData = [0 7 27 32 52 57 77 82 102 107 127 132 157 187 200]
      | sbobj.Groups(5).Signals(3).YData = [0 5 5 10 10 15 15 20 20 25 25 30 30 0 0]
      | sbobj.Groups(5).TimeRange = [0 200]
  Z : Outport
  X : Outport  Tag=STV Outport  Port=2
  Y : Outport  Tag=STV Outport  Port=3
  wires:
  Demux/1 -> Z/1
  FromWs/1 -> Demux/1
  Demux/2 -> X/1
  Demux/3 -> Y/1

== system bh_6dof_quat_integrate/CONT_SYS Force_Moment_CMDS/FM_CMD_LIMITS ==
  T_CMD : Inport
  TQ_Roll : Inport  Port=2
  TQ_Pitch : Inport  Port=3
  TQ_Yaw : Inport  Port=4
  Mux : Mux
  Saturation : Saturate  UpperLimit=4*P_one_prop.thrust_max  LowerLimit=0
      settings: AttributesFormatString=|
      | MAX =    %<UpperLimit>
      | MIN = %<LowerLimit>
  Saturation1 : Saturate  UpperLimit=2*P_one_prop.TQ_max  LowerLimit=-2*P_one_prop.TQ_max
      settings: AttributesFormatString=|
      | MAX =    %<UpperLimit>
      | MIN = %<LowerLimit>
  Saturation2 : Saturate  UpperLimit="P_one_prop.thrust_max *  P_veh.L_CG_to_mot"  LowerLimit="-P_one_prop.thrust_max *  P_veh.L_CG_to_mot"
      settings: AttributesFormatString=|
      | MAX =    %<UpperLimit>
      | MIN = %<LowerLimit>
  Saturation3 : Saturate  UpperLimit="P_one_prop.thrust_max *  P_veh.L_CG_to_mot"  LowerLimit="-P_one_prop.thrust_max *  P_veh.L_CG_to_mot"
      settings: AttributesFormatString=|
      | MAX =    %<UpperLimit>
      | MIN = %<LowerLimit>
  THRUST : Outport
  TQ_Roll_X : Outport  Port=2
  TQ_Pitch_Y : Outport  Port=3
  TQ_Yaw_Z : Outport  Port=4
  CMD_VEC : Outport  Port=5
  wires:
  TQ_Yaw/1 -> Saturation1/1
  T_CMD/1 -> Saturation/1
  TQ_Pitch/1 -> Saturation2/1
  TQ_Roll/1 -> Saturation3/1
  Saturation/1 -> [THRUST], THRUST/1
  Saturation3/1 -> [TQ_Roll_X], TQ_Roll_X/1
  Saturation2/1 -> [TQ_Pitch_Y], TQ_Pitch_Y/1
  Saturation1/1 -> [TQ_Yaw_Z], TQ_Yaw_Z/1
  Mux/1 -> CMD_VEC/1
  [THRUST] -> Mux/1
  [TQ_Roll_X] -> Mux/2
  [TQ_Pitch_Y] -> Mux/3
  [TQ_Yaw_Z] -> Mux/4

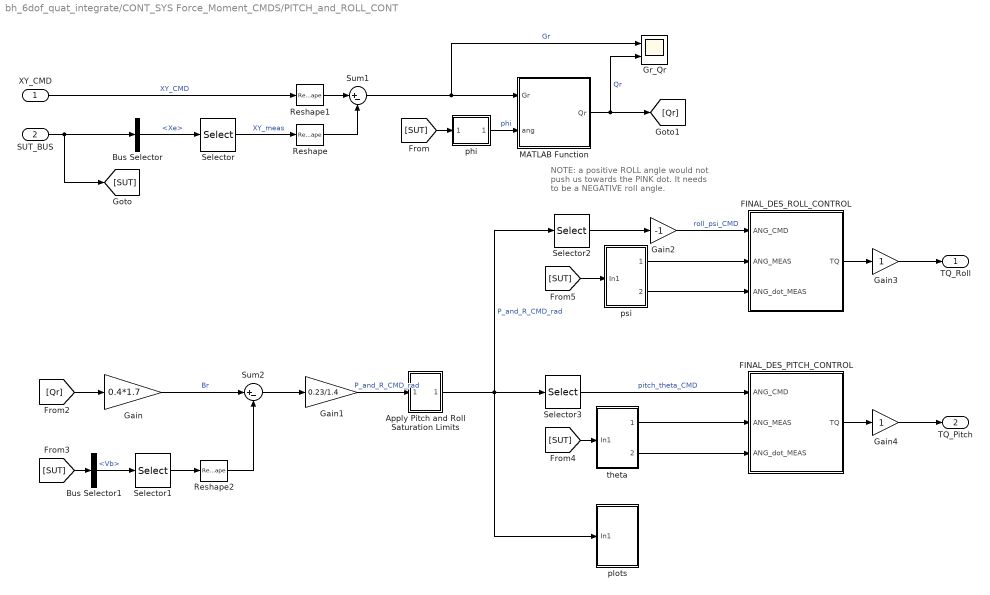
== system bh_6dof_quat_integrate/CONT_SYS Force_Moment_CMDS/PITCH_and_ROLL_CONT ==
  note: NOTE:  a positive ROLL angle would
      | not push us towards the PINK dot.  It
      | needs to be a NEGATIVE roll angle.
  XY_CMD : Inport
  SUT_BUS : Inport  Port=2
  Apply Pitch and Roll Saturation Limits : Subsystem
  Bus Selector : BusSelector  OutputSignals=Xe
  Bus Selector1 : BusSelector  OutputSignals=Vb
  FINAL_DES_PITCH_CONTROL : Subsystem
  FINAL_DES_ROLL_CONTROL : Subsystem
  Gain : Gain  Gain=0.4*1.7
  Gain1 : Gain  Gain=0.23/1.4
  Gain2 : Gain  Gain=-1
  Gain3 : Gain
  Gain4 : Gain
  Gr_Qr : Scope  NumInputPorts=2
  MATLAB Function : MATLAB Function  TreatAsAtomicUnit=on
  Reshape : Reshape  OutputDimensionality=Column vector (2-D)
  Reshape1 : Reshape  OutputDimensionality=Column vector (2-D)
  Reshape2 : Reshape  OutputDimensionality=Column vector (2-D)
  Selector : Selector  InputPortWidth=3  IndexOptions=Index vector (dialog)  Indices=[1 2]  OutputSizes=1
  Selector1 : Selector  InputPortWidth=3  IndexOptions=Index vector (dialog)  Indices=[1 2]  OutputSizes=1
  Selector2 : Selector  InputPortWidth=2  IndexOptions=Index vector (dialog)  Indices=2  OutputSizes=1
  Selector3 : Selector  InputPortWidth=2  IndexOptions=Index vector (dialog)  Indices=1  OutputSizes=1
  Sum1 : Sum  Inputs=|+-
  Sum2 : Sum  Inputs=|+-
  phi : Subsystem
  plots : Subsystem
  psi : Subsystem
  theta : Subsystem
  TQ_Roll : Outport
  TQ_Pitch : Outport  Port=2
  wires:
  Bus Selector/1 -> Selector/1  "<Xe>"
  Selector/1 -> Reshape/1  "XY_meas"
  SUT_BUS/1 -> Bus Selector/1, [SUT]
  XY_CMD/1 -> Reshape1/1  "XY_CMD"
  Reshape1/1 -> Sum1/1
  Reshape/1 -> Sum1/2
  Sum1/1 -> Gr_Qr/1, MATLAB Function/1(Gr)  "Gr"
  [SUT] -> phi/1(In1)
  phi/1(Out1) -> MATLAB Function/2(ang)  "phi"
  MATLAB Function/1(Qr) -> Gr_Qr/2, [Qr]  "Qr"
  [Qr] -> Gain/1
  Gain/1 -> Sum2/1  "Br"
  Bus Selector1/1 -> Selector1/1  "<Vb>"
  [SUT] -> Bus Selector1/1
  Selector1/1 -> Reshape2/1
  Reshape2/1 -> Sum2/2
  Sum2/1 -> Gain1/1
  [SUT] -> theta/1(In1)
  theta/1(Out1) -> FINAL_DES_PITCH_CONTROL/2(ANG_MEAS)
  theta/2(Out2) -> FINAL_DES_PITCH_CONTROL/3(ANG_dot_MEAS)
  Selector3/1 -> FINAL_DES_PITCH_CONTROL/1(ANG_CMD)  "pitch_theta_CMD"
  FINAL_DES_PITCH_CONTROL/1(TQ) -> Gain4/1
  Gain1/1 -> Apply Pitch and Roll Saturation Limits/1(In1)  "P_and_R_CMD_rad"
  Selector2/1 -> Gain2/1
  psi/1(Out1) -> FINAL_DES_ROLL_CONTROL/2(ANG_MEAS)
  psi/2(Out2) -> FINAL_DES_ROLL_CONTROL/3(ANG_dot_MEAS)
  [SUT] -> psi/1(In1)
  FINAL_DES_ROLL_CONTROL/1(TQ) -> Gain3/1
  Gain2/1 -> FINAL_DES_ROLL_CONTROL/1(ANG_CMD)  "roll_psi_CMD"
  Apply Pitch and Roll Saturation Limits/1(Out1) -> plots/1(In1), Selector3/1, Selector2/1  "P_and_R_CMD_rad"
  Gain3/1 -> TQ_Roll/1
  Gain4/1 -> TQ_Pitch/1

== system bh_6dof_quat_integrate/CONT_SYS Force_Moment_CMDS/YAW_CONT ==
  Yaw_CMD : Inport
  SUT_BUS : Inport  Port=2
  Bus Selector3 : BusSelector  OutputSignals=phi; theta; psi
  Bus Selector4 : BusSelector  OutputSignals=dphi; dtheta; dpsi
  FINAL_DES_YAW_CONTROL_SYSTEM : Subsystem
  Selector2 : Selector  InputPortWidth=3  IndexOptions=Index vector (dialog)  Indices=1  OutputSizes=1
  Selector3 : Selector  InputPortWidth=3  IndexOptions=Index vector (dialog)  Indices=1  OutputSizes=1
  TQ_Yaw : Outport
  wires:
  Selector2/1 -> FINAL_DES_YAW_CONTROL_SYSTEM/2(YAW_MEAS)
  Yaw_CMD/1 -> FINAL_DES_YAW_CONTROL_SYSTEM/1(YAW_CMD)
  Selector3/1 -> FINAL_DES_YAW_CONTROL_SYSTEM/3(YAW_dot_MEAS)
  FINAL_DES_YAW_CONTROL_SYSTEM/1(TQ_YAW) -> TQ_Yaw/1  "TQ_Z_YAW"
  Bus Selector4/1 -> Selector3/1  "<dphi; dtheta; dpsi>"
  Bus Selector3/1 -> Selector2/1  "<phi; theta; psi>"
  SUT_BUS/1 -> Bus Selector4/1, Bus Selector3/1

== system bh_6dof_quat_integrate/CONT_SYS Force_Moment_CMDS/Z_CONT ==
  Ze_CMD : Inport
  SUT_BUS : Inport  Port=2
  Bus Selector : BusSelector  OutputSignals=Xe
  Bus Selector2 : BusSelector  OutputSignals=Ve
  FINAl_DES_ALTITUDE_CONTROL_SYSTEM : Subsystem
  Selector : Selector  InputPortWidth=3  IndexOptions=Index vector (dialog)  Indices=3  OutputSizes=1
  Selector1 : Selector  InputPortWidth=3  IndexOptions=Index vector (dialog)  Indices=3  OutputSizes=1
  Ze_to_Altitude : bh_6dof_LIBRARY/MODELS/Ze_to_Altitude  SystemSampleTime=-1  Latency=0  AutoFrameSizeCalculation=off
  THRUST : Outport
  wires:
  Selector1/1 -> FINAl_DES_ALTITUDE_CONTROL_SYSTEM/3(Ze_dot_MEAS)
  Ze_to_Altitude/1 -> FINAl_DES_ALTITUDE_CONTROL_SYSTEM/2(Ze_MEAS)
  FINAl_DES_ALTITUDE_CONTROL_SYSTEM/1(THRUST) -> THRUST/1
  SUT_BUS/1 -> Bus Selector2/1, Bus Selector/1
  Ze_CMD/1 -> FINAl_DES_ALTITUDE_CONTROL_SYSTEM/1(Ze_CMD)
  Bus Selector2/1 -> Selector1/1  "<Ve>"
  Bus Selector/1 -> Selector/1  "<Xe>"
  Selector/1 -> Ze_to_Altitude/1

== system bh_6dof_quat_integrate/CONT_SYS W_MOT_CMDS/MOTOR_sys ==
  w_CMD : Inport
  Demux : Demux
  MOTOR_1 : Subsystem
      mask Display: image('bh_PIC_MOTOR.jpg');
  MOTOR_2 : Subsystem
      mask Display: image('bh_PIC_MOTOR.jpg');
  MOTOR_3 : Subsystem
      mask Display: image('bh_PIC_MOTOR.jpg');
  MOTOR_4 : Subsystem
      mask Display: image('bh_PIC_MOTOR.jpg');
  Mux : Mux
  w CMD vs Actual : Scope  NumInputPorts=4
  w_MUX : Subsystem
  w : Outport
  wires:
  MOTOR_4/1(w) -> Mux/4
  MOTOR_3/1(w) -> Mux/3
  MOTOR_2/1(w) -> Mux/2
  MOTOR_1/1(w) -> Mux/1
  Demux/1 -> MOTOR_1/1(w_CMD)
  Demux/2 -> MOTOR_2/1(w_CMD)
  Demux/3 -> MOTOR_3/1(w_CMD)
  Demux/4 -> MOTOR_4/1(w_CMD)
  w_CMD/1 -> [W_CMD], Demux/1
  Mux/1 -> [W], w/1
  w_MUX/4(w4) -> w CMD vs Actual/4
  w_MUX/2(w2) -> w CMD vs Actual/2
  w_MUX/3(w3) -> w CMD vs Actual/3
  w_MUX/1(w1) -> w CMD vs Actual/1
  [W_CMD] -> w_MUX/1(W_CMD)
  [W] -> w_MUX/2(W)

== system bh_6dof_quat_integrate/CONT_SYS W_MOT_CMDS/SIGN_CONVENTIONS ==

== system bh_6dof_quat_integrate/CONT_SYS W_MOT_CMDS/W2_checker ==
  w2_CMD : Inport
  Assertion{,1..3} (4 alike) : Assertion
  Compare To Constant : simulink/Logic and Bit Operations/Compare To Constant  relop=>=  const=0  OutDataTypeStr=boolean
  Demux : Demux
  w2 : Outport
  wires:
  w2_CMD/1 -> w2/1, Compare To Constant/1
  Compare To Constant/1 -> Demux/1
  Demux/1 -> Assertion/1
  Demux/4 -> Assertion3/1
  Demux/3 -> Assertion2/1
  Demux/2 -> Assertion1/1

== system bh_6dof_quat_integrate/Construct_Fb_VECTOR/Gravity_G_to_B ==
  note: F_B = ^BR_G * F_G
  bRg : Inport
  Constant : Constant  Value=P_veh.mass
  Fg_gravity : Constant  Value=[0;0;-9.81]  VectorParams1D=off
  Product : Product  Multiplication=Matrix(*)
  Product1 : Product
  Fb_gravity : Outport
  wires:
  bRg/1 -> Product/1
  Product/1 -> Fb_gravity/1  "Fb"
  Product1/1 -> Product/2  "m*g"
  Fg_gravity/1 -> Product1/1  "Fg"
  Constant/1 -> Product1/2

== system bh_6dof_quat_integrate/FM_EYES/FM_Mux ==
  FM_CMD : Inport
  FM : Inport  Port=2
  Demux1 : Demux
  Demux2 : Demux
  Mux{,1..3} (4 alike) : Mux  Inputs=2
  Y1 : Outport
  Y2 : Outport  Port=2
  w3 : Outport  Port=3
  Y4 : Outport  Port=4
  wires:
  FM_CMD/1 -> Demux2/1
  FM/1 -> Demux1/1
  Mux/1 -> Y1/1
  Mux1/1 -> Y2/1
  Mux3/1 -> Y4/1
  Mux2/1 -> w3/1
  Demux2/1 -> Mux/1
  Demux2/2 -> Mux1/1
  Demux2/3 -> Mux2/1
  Demux2/4 -> Mux3/1
  Demux1/1 -> Mux/2
  Demux1/2 -> Mux1/2
  Demux1/3 -> Mux2/2
  Demux1/4 -> Mux3/2

== system bh_6dof_quat_integrate/FM_EYES/SIGN_CONVENTIONS ==

== system bh_6dof_quat_integrate/Gyroscopic moments/Apply SIGN to w_motor ==
  w_mot_UN : Inport
  Demux : Demux
  Gain : Gain  Gain=-1
  Gain1 : Gain  Gain=-1
  Mux : Mux
  Reshape1 : Reshape  OutputDimensionality=Column vector (2-D)
  w_mot_signed : Outport
  wires:
  w_mot_UN/1 -> Demux/1
  Demux/2 -> Gain/1
  Demux/4 -> Gain1/1
  Gain/1 -> Mux/2
  Gain1/1 -> Mux/4
  Demux/3 -> Mux/3
  Demux/1 -> Mux/1
  Mux/1 -> Reshape1/1
  Reshape1/1 -> w_mot_signed/1

== system bh_6dof_quat_integrate/Gyroscopic moments/EYES ==
  M1 : Inport
  M2 : Inport  Port=2
  M3 : Inport  Port=3
  M4 : Inport  Port=4
  MT : Inport  Port=5
  Demux{,1..4} (5 alike) : Demux  Outputs=3
  M1_to_M4 : Scope  NumInputPorts=12
  M_TOTAL : Scope  NumInputPorts=3
  wires:
  Demux/1 -> M1_to_M4/1  "M1_X"
  Demux/2 -> M1_to_M4/2  "M1_Y"
  Demux/3 -> M1_to_M4/3  "M1_Z"
  Demux1/3 -> M1_to_M4/6  "M2_Z"
  Demux1/2 -> M1_to_M4/5  "M2_Y"
  Demux1/1 -> M1_to_M4/4  "M2_X"
  Demux2/1 -> M1_to_M4/7  "M3_X"
  Demux2/2 -> M1_to_M4/8  "M3_Y"
  Demux2/3 -> M1_to_M4/9  "M3_Z"
  Demux3/1 -> M1_to_M4/10  "M4_X"
  Demux3/2 -> M1_to_M4/11  "M4_Y"
  Demux3/3 -> M1_to_M4/12  "M4_Z"
  M1/1 -> Demux/1
  M2/1 -> Demux1/1
  M3/1 -> Demux2/1
  M4/1 -> Demux3/1
  MT/1 -> Demux4/1
  Demux4/1 -> M_TOTAL/1  "M_TOTAL_X"
  Demux4/2 -> M_TOTAL/2  "M_TOTAL_Y"
  Demux4/3 -> M_TOTAL/3  "M_TOTAL_Z"

== system bh_6dof_quat_integrate/Gyroscopic moments/GYROSCOPIC moments ==
  note: \omega_y * I_{zz} * \Omega_z
      |
      | -1*\omega_x * I_{zz} * \Omega_z
      |
      | I_{zz} * \Omega_z^'
  Izz_mot_prop : Inport
  wb_veh_vec : Inport  Port=2
  w_mot_signed : Inport  Port=3
  dwdt_motor : Inport  Port=4
  Gain : Gain  Gain=-1
  Gain1 : Gain  Gain=-1
  Mux : Mux  Inputs=3
  Product : Product
  Product1 : Product  Inputs=3
  Product2 : Product  Inputs=3
  Reshape : Reshape  OutputDimensionality=Column vector (2-D)
  Selector : Selector  InputPortWidth=3  IndexOptions=Index vector (dialog)  Indices=2  OutputSizes=1
  Selector1 : Selector  InputPortWidth=3  IndexOptions=Index vector (dialog)  Indices=1  OutputSizes=1
  add_to_Mb : Outport
  wires:
  Mux/1 -> Reshape/1
  Reshape/1 -> Gain1/1
  Product2/1 -> Gain/1
  Product1/1 -> Mux/1
  Product/1 -> Mux/3
  dwdt_motor/1 -> Product/2  "dwdt_mot_prop"
  [Izz] -> Product/1
  [Izz] -> Product2/3
  Selector1/1 -> Product2/2  "wx"
  w_mot_signed/1 -> Product1/3, Product2/1  "w_mot_prop"
  [Izz] -> Product1/1
  Selector/1 -> Product1/2  "wy"
  Izz_mot_prop/1 -> [Izz]
  wb_veh_vec/1 -> Selector/1, Selector1/1
  Gain/1 -> Mux/2
  Gain1/1 -> add_to_Mb/1

== system bh_6dof_quat_integrate/Gyroscopic moments/GYROSCOPIC moments1 ==
  note: \omega_y * I_{zz} * \Omega_z
      |
      | -1*\omega_x * I_{zz} * \Omega_z
      |
      | I_{zz} * \Omega_z^'
  Izz_mot_prop : Inport
  wb_veh_vec : Inport  Port=2
  w_mot_signed : Inport  Port=3
  dwdt_motor : Inport  Port=4
  Gain : Gain  Gain=-1
  Gain1 : Gain  Gain=-1
  Mux : Mux  Inputs=3
  Product : Product
  Product1 : Product  Inputs=3
  Product2 : Product  Inputs=3
  Reshape : Reshape  OutputDimensionality=Column vector (2-D)
  Selector : Selector  InputPortWidth=3  IndexOptions=Index vector (dialog)  Indices=2  OutputSizes=1
  Selector1 : Selector  InputPortWidth=3  IndexOptions=Index vector (dialog)  Indices=1  OutputSizes=1
  add_to_Mb : Outport
  wires:
  Mux/1 -> Reshape/1
  Reshape/1 -> Gain1/1
  Product2/1 -> Gain/1
  Product1/1 -> Mux/1
  Product/1 -> Mux/3
  dwdt_motor/1 -> Product/2  "dwdt_mot_prop"
  [Izz] -> Product/1
  [Izz] -> Product2/3
  Selector1/1 -> Product2/2  "wx"
  w_mot_signed/1 -> Product1/3, Product2/1  "w_mot_prop"
  [Izz] -> Product1/1
  Selector/1 -> Product1/2  "wy"
  Izz_mot_prop/1 -> [Izz]
  wb_veh_vec/1 -> Selector/1, Selector1/1
  Gain/1 -> Mux/2
  Gain1/1 -> add_to_Mb/1

== system bh_6dof_quat_integrate/Gyroscopic moments/GYROSCOPIC moments2 ==
  note: \omega_y * I_{zz} * \Omega_z
      |
      | -1*\omega_x * I_{zz} * \Omega_z
      |
      | I_{zz} * \Omega_z^'
  Izz_mot_prop : Inport
  wb_veh_vec : Inport  Port=2
  w_mot_signed : Inport  Port=3
  dwdt_motor : Inport  Port=4
  Gain : Gain  Gain=-1
  Gain1 : Gain  Gain=-1
  Mux : Mux  Inputs=3
  Product : Product
  Product1 : Product  Inputs=3
  Product2 : Product  Inputs=3
  Reshape : Reshape  OutputDimensionality=Column vector (2-D)
  Selector : Selector  InputPortWidth=3  IndexOptions=Index vector (dialog)  Indices=2  OutputSizes=1
  Selector1 : Selector  InputPortWidth=3  IndexOptions=Index vector (dialog)  Indices=1  OutputSizes=1
  add_to_Mb : Outport
  wires:
  Mux/1 -> Reshape/1
  Reshape/1 -> Gain1/1
  Product2/1 -> Gain/1
  Product1/1 -> Mux/1
  Product/1 -> Mux/3
  dwdt_motor/1 -> Product/2  "dwdt_mot_prop"
  [Izz] -> Product/1
  [Izz] -> Product2/3
  Selector1/1 -> Product2/2  "wx"
  w_mot_signed/1 -> Product1/3, Product2/1  "w_mot_prop"
  [Izz] -> Product1/1
  Selector/1 -> Product1/2  "wy"
  Izz_mot_prop/1 -> [Izz]
  wb_veh_vec/1 -> Selector/1, Selector1/1
  Gain/1 -> Mux/2
  Gain1/1 -> add_to_Mb/1

== system bh_6dof_quat_integrate/Gyroscopic moments/GYROSCOPIC moments3 ==
  note: \omega_y * I_{zz} * \Omega_z
      |
      | -1*\omega_x * I_{zz} * \Omega_z
      |
      | I_{zz} * \Omega_z^'
  Izz_mot_prop : Inport
  wb_veh_vec : Inport  Port=2
  w_mot_signed : Inport  Port=3
  dwdt_motor : Inport  Port=4
  Gain : Gain  Gain=-1
  Gain1 : Gain  Gain=-1
  Mux : Mux  Inputs=3
  Product : Product
  Product1 : Product  Inputs=3
  Product2 : Product  Inputs=3
  Reshape : Reshape  OutputDimensionality=Column vector (2-D)
  Selector : Selector  InputPortWidth=3  IndexOptions=Index vector (dialog)  Indices=2  OutputSizes=1
  Selector1 : Selector  InputPortWidth=3  IndexOptions=Index vector (dialog)  Indices=1  OutputSizes=1
  add_to_Mb : Outport
  wires:
  Mux/1 -> Reshape/1
  Reshape/1 -> Gain1/1
  Product2/1 -> Gain/1
  Product1/1 -> Mux/1
  Product/1 -> Mux/3
  dwdt_motor/1 -> Product/2  "dwdt_mot_prop"
  [Izz] -> Product/1
  [Izz] -> Product2/3
  Selector1/1 -> Product2/2  "wx"
  w_mot_signed/1 -> Product1/3, Product2/1  "w_mot_prop"
  [Izz] -> Product1/1
  Selector/1 -> Product1/2  "wy"
  Izz_mot_prop/1 -> [Izz]
  wb_veh_vec/1 -> Selector/1, Selector1/1
  Gain/1 -> Mux/2
  Gain1/1 -> add_to_Mb/1

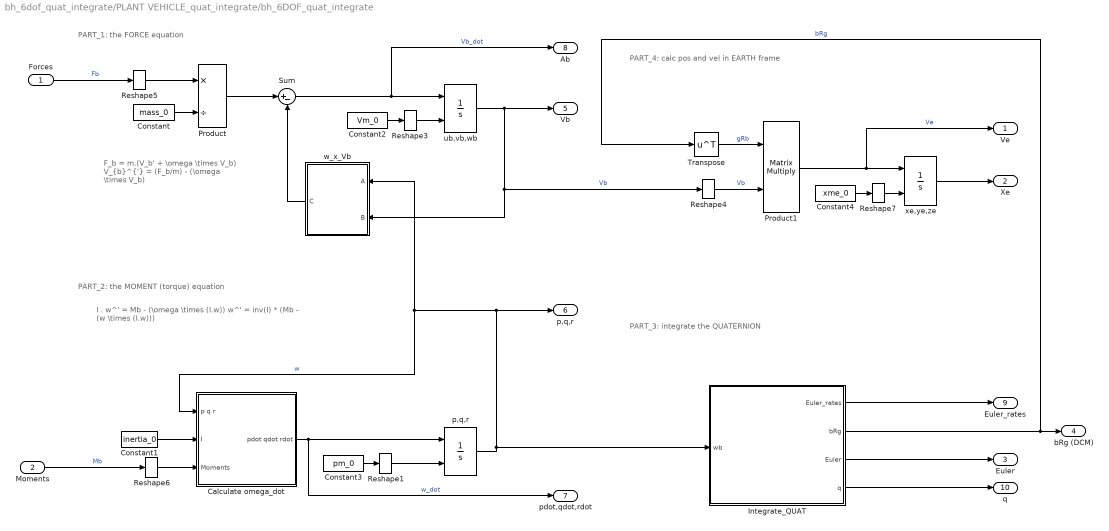
== system bh_6dof_quat_integrate/PLANT VEHICLE_quat_integrate/bh_6DOF_quat_integrate ==
  note: PART_4: calc pos and vel in EARTH frame
  note: PART_3: integrate the QUATERNION
  note: PART_2: the MOMENT (torque) equation
  note: PART_1: the FORCE equation
  note: F_b = m.(V_b' + \omega \times V_b)
      |
      | V_{b}^{'} = (F_b/m) - (\omega \times V_b)
  note: I . w^' = Mb - (\omega \times (I.w))
      |
      | w^' = inv(I) * (Mb - (w \times (I.w)))
  Forces : Inport
  Moments : Inport  Port=2
  Calculate omega_dot : Subsystem
  Constant : Constant  Value=mass_0  OutDataTypeStr=Inherit: Inherit via back propagation
  Constant1 : Constant  Value=inertia_0  OutDataTypeStr=Inherit: Inherit via back propagation
  Constant2 : Constant  Value=Vm_0  OutDataTypeStr=Inherit: Inherit via back propagation
  Constant3 : Constant  Value=pm_0  OutDataTypeStr=Inherit: Inherit via back propagation
  Constant4 : Constant  Value=xme_0  OutDataTypeStr=Inherit: Inherit via back propagation
  Integrate_QUAT : Subsystem
  Product : Product  Inputs=*/  SaturateOnIntegerOverflow=on  OutDataTypeStr=Inherit: Same as first input
  Product1 : Product  Multiplication=Matrix(*)  SaturateOnIntegerOverflow=on  InputSameDT=on  OutDataTypeStr=Inherit: Same as first input
  Reshape{1,3..7} (6 alike) : Reshape  OutputDimensionality=Column vector (2-D)
  Sum : Sum  Inputs=|+-  SaturateOnIntegerOverflow=on
  Transpose : Math  Operator=transpose  SaturateOnIntegerOverflow=on
  "p,q,r " : Integrator  InitialConditionSource=external  InitialCondition=pm_0
  ub,vb,wb : Integrator  InitialConditionSource=external  InitialCondition=Vm_0
  w_x_Vb : Subsystem
      mask Display:
      | text(.5,.5,'Cross\nProduct\n\nC = AxB', ...
      | 	'HorizontalAlignment','Center',...
      | 	'VerticalAlignment','middle')
  xe,ye,ze : Integrator  InitialConditionSource=external  InitialCondition=xme_0
  Ve : Outport
  Xe : Outport  Port=2
  Euler : Outport  Port=3
  bRg (DCM) : Outport  Port=4
  Vb : Outport  Port=5
  p,q,r : Outport  Port=6
  pdot,qdot,rdot : Outport  Port=7
  Ab : Outport  Port=8
  Euler_rates : Outport  Port=9
  q : Outport  Port=10
  wires:
  Integrate_QUAT/3(Euler) -> Euler/1
  Integrate_QUAT/1(Euler_rates) -> Euler_rates/1
  Constant4/1 -> Reshape7/1
  Reshape7/1 -> xe,ye,ze/2
  Product1/1 -> xe,ye,ze/1, Ve/1  "Ve"
  Constant3/1 -> Reshape1/1
  Reshape1/1 -> "p,q,r "/2
  Reshape6/1 -> Calculate omega_dot/3(Moments)
  Reshape5/1 -> Product/1
  Reshape3/1 -> ub,vb,wb/2
  Constant2/1 -> Reshape3/1
  Calculate omega_dot/1(pdot qdot rdot) -> "p,q,r "/1, pdot,qdot,rdot/1  "w_dot"
  Reshape4/1 -> Product1/2  "Vb"
  Transpose/1 -> Product1/1  "gRb"
  Constant1/1 -> Calculate omega_dot/2(I)
  w_x_Vb/1(C) -> Sum/2
  xe,ye,ze/1 -> Xe/1
  "p,q,r "/1 -> w_x_Vb/1(A), Calculate omega_dot/1(p q r), p,q,r/1, Integrate_QUAT/1(wb)  "w"
  Moments/1 -> Reshape6/1  "Mb"
  Product/1 -> Sum/1
  Constant/1 -> Product/2
  Forces/1 -> Reshape5/1  "Fb"
  ub,vb,wb/1 -> Vb/1, w_x_Vb/2(B), Reshape4/1  "Vb"
  Sum/1 -> ub,vb,wb/1, Ab/1  "Vb_dot"
  Integrate_QUAT/2(bRg) -> Transpose/1, bRg (DCM)/1  "bRg"
  Integrate_QUAT/4(q) -> q/1

== system bh_6dof_quat_integrate/XYZ CMD_LIMITS/prefilter ==
  note: Y = U *     wn^2/( s^2 + 2*p*wn*s + wn^2)
      | Y*( s^2 + 2*p*wn*s + wn^2) = U * wn^2
      |
      | y'' + y'*2*p*wn + y*wn^2 = U*wn^2
  U : Inport
  Gain : Gain  Gain=2*p*wn
  Gain1 : Gain  Gain=wn^2
  Gain2 : Gain  Gain=wn^2
  Integrator : Integrator
  Integrator1 : Integrator
  Sum : Sum  Inputs=|+--
  U_filt : Outport
  U_DOT : Outport  Port=2
  wires:
  Integrator/1 -> Integrator1/1, [Y_DOT], Gain/1  "y_dot"
  Sum/1 -> Integrator/1  "y_dot_dot"
  Integrator1/1 -> Gain1/1, U_filt/1  "y"
  U/1 -> Gain2/1
  Gain2/1 -> Sum/1
  Gain/1 -> Sum/3
  Gain1/1 -> Sum/2
  [Y_DOT] -> U_DOT/1

== system bh_6dof_quat_integrate/CONT_SYS Force_Moment_CMDS/PITCH_and_ROLL_CONT/Apply Pitch and Roll Saturation Limits ==
  In1 : Inport
  Degrees to Radians : simulink_extras/Transformations/Degrees to Radians
  Radians to Degrees : simulink_extras/Transformations/Radians to Degrees
  Saturation : Saturate  UpperLimit=P_veh.LIMITS_tilt_max_deg  LowerLimit=-1*P_veh.LIMITS_tilt_max_deg
      settings: AttributesFormatString=|
      | MAX =    %<UpperLimit>
      | MIN = %<LowerLimit>
  Out1 : Outport
  wires:
  In1/1 -> Radians to Degrees/1
  Saturation/1 -> Degrees to Radians/1
  Radians to Degrees/1 -> Saturation/1
  Degrees to Radians/1 -> Out1/1
